simulink model "bandpass"  (R2016a)
settings: Solver=VariableStepAuto  StartTime=0.0  StopTime=5.5  RelTol=1e-3
undefined symbols (not defined in the file): fdesignblkfcn, gcbh
libraries: dspvision x4
(part 1 of 4)
settings Model: Creator=soup  LastModifiedBy=soup

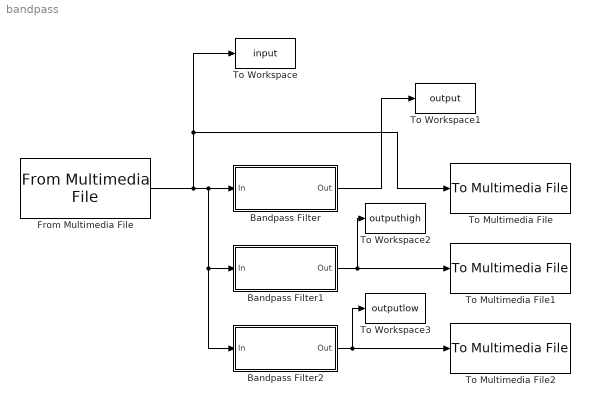
== system bandpass ==
  Bandpass Filter : Subsystem  DialogController=fdesignblkfcn  InitFcn=fdesignblkfcn(gcbh, {'InitFcn'});  mask(Bandpass Filter){}
      mask help: Design a bandpass filter
      settings: CopyFcn=fdesignblkfcn(gcbh, {'CopyFcn'});
      mask Help: helpview(mapfilelocation('dsp'), 'dspbandpassfilter');
      mask Display: disp('Bandpass');
  Bandpass Filter1 : Subsystem  DialogController=fdesignblkfcn  InitFcn=fdesignblkfcn(gcbh, {'InitFcn'});  mask(Bandpass Filter){}
      mask help: Design a bandpass filter
      settings: CopyFcn=fdesignblkfcn(gcbh, {'CopyFcn'});
      mask Help: helpview(mapfilelocation('dsp'), 'dspbandpassfilter');
      mask Display: disp('Bandpass');
  Bandpass Filter2 : Subsystem  DialogController=fdesignblkfcn  InitFcn=fdesignblkfcn(gcbh, {'InitFcn'});  mask(Bandpass Filter){}
      mask help: Design a bandpass filter
      settings: CopyFcn=fdesignblkfcn(gcbh, {'CopyFcn'});
      mask Help: helpview(mapfilelocation('dsp'), 'dspbandpassfilter');
      mask Display: disp('Bandpass');
  From Multimedia File : dspvision/From Multimedia File  inputFilename=C:\Users\soup\Videos\Captures\vlc-record-2016-11-03-13h30m58s-OutsideF.m4a-.mp4  loop=on  numPlays=1  outputStreams=Audio only  videoDataType=single  audioDataType=double  inheritSampleTime=on  userDefinedSampleTime=1/30  noAudioOutput=off  isIntensityVideo=off  fourcc=RGB  colorVideoFormat=Separate color signals  outputEOF=off  dataOrg=Column-major  audioFrameSize=1024  computeAudioFrameSize=off  outSamplingMode=Sample based
  To Multimedia File : dspvision/To Multimedia File  outputFilename=C:\Users\soup\Dropbox (MIT)\Orange Team\Electrical\Sound Files 10_31_16\derpin.wav  streamSelection=Audio only  videoCompressor=None (uncompressed)  audioCompressor=None (uncompressed)  imagePorts=Separate color signals  fileType=WAV  audioDatatype=16-bit integer  fourcc=RGB  videoQuality=75  mj2000CompFactor=10
  To Multimedia File1 : dspvision/To Multimedia File  outputFilename=C:\Users\soup\Dropbox (MIT)\Orange Team\Electrical\Sound Files 10_31_16\derpouthigh.wav  streamSelection=Audio only  videoCompressor=None (uncompressed)  audioCompressor=None (uncompressed)  imagePorts=Separate color signals  fileType=WAV  audioDatatype=16-bit integer  fourcc=RGB  videoQuality=75  mj2000CompFactor=10
  To Multimedia File2 : dspvision/To Multimedia File  outputFilename=C:\Users\soup\Dropbox (MIT)\Orange Team\Electrical\Sound Files 10_31_16\derpoutlow.wav  streamSelection=Audio only  videoCompressor=None (uncompressed)  audioCompressor=None (uncompressed)  imagePorts=Separate color signals  fileType=WAV  audioDatatype=16-bit integer  fourcc=RGB  videoQuality=75  mj2000CompFactor=10
  To Workspace : ToWorkspace  VariableName=input  SaveFormat=Timeseries  SampleTime=-1
      settings: Save2DSignal=2-D array (concatenate along first dimension)
  To Workspace1 : ToWorkspace  VariableName=output  SaveFormat=Timeseries  SampleTime=-1
      settings: Save2DSignal=2-D array (concatenate along first dimension)
  To Workspace2 : ToWorkspace  VariableName=outputhigh  SaveFormat=Timeseries  SampleTime=-1
      settings: Save2DSignal=2-D array (concatenate along first dimension)
  To Workspace3 : ToWorkspace  VariableName=outputlow  SaveFormat=Timeseries  SampleTime=-1
      settings: Save2DSignal=2-D array (concatenate along first dimension)
  wires:
  From Multimedia File/1 -> Bandpass Filter2/1(In), Bandpass Filter1/1(In), Bandpass Filter/1(In), To Workspace/1, To Multimedia File/1
  Bandpass Filter/1(Out) -> To Workspace1/1
  Bandpass Filter1/1(Out) -> To Workspace2/1, To Multimedia File1/1
  Bandpass Filter2/1(Out) -> To Workspace3/1, To Multimedia File2/1
